simulink model "DCMachine"  (R2020a)
settings: Solver=VariableStepAuto  StartTime=0.0  StopTime=10.0  RelTol=1e-3
libraries: powerlib x4
settings Model: Creator=royde  LastModifiedBy=royde

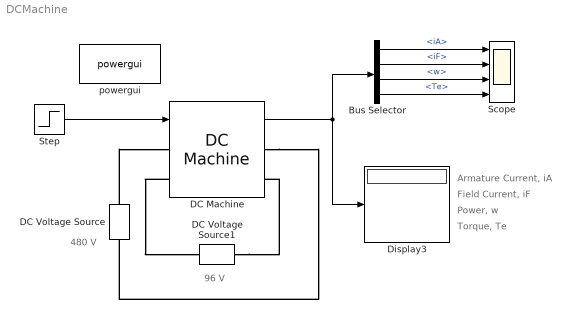
== system DCMachine ==
  note: Power, w
  note: Field Current, iF
  note: Armature Current, iA
  note: Torque, Te
  note: 96 V
  note: 480 V
  Bus Selector : BusSelector  OutputSignals=iA,iF,w,Te
  DC Machine : powerlib/Machines/DC Machine  PresetModel=03: 5HP 500V 1750RPM Field:300V  MechanicalLoad=Torque TL  FieldType=Wound  ShowDetailedParameters=on  MeasurementBus=on  RLa=[11.2 0.1215]  RLf=[281.3 156]  Laf=1.976  MachineConstant=Torque constant (N.m/A)  Ke=1.8  Kt=1.8  J=0.02215  Bm=0.002953  Tf=0.5161  w0=1  Ifinit=0.341272662637753  TsPowergui=0  TsBlock=-1
  DC Voltage Source : powerlib/Electrical Sources/DC Voltage Source  Amplitude=480  Measurements=None
  DC Voltage Source1 : powerlib/Electrical Sources/DC Voltage Source  Amplitude=96  Measurements=Voltage
  Display3 : Display
  Scope : Scope  NumInputPorts=4
  Step : Step  SampleTime=0
  powergui : powerlib/powergui  Priority=1  SimulationMode=Continuous  SampleTime=50e-6  frequency=60  Iterations=50  frequencyindice=0  Pbase=100e6  ErrMax=1e-4  UnitsV=kV  UnitsW=MW  buscounter=0  FunctionMessages=off  echomessages=off  EnableUseOfTLC=off  CurrentSourceSwitches=off  DisableSnubberDevices=off  DisableRonSwitches=off  DisableVfSwitches=off  DisplayEquations=off  AutomaticDiscreteSolvers=off  SolverType=Tustin/Backward Euler (TBE)  Interpol=off  ExternalGateDelay=off  methode=off  Ts=100  x0status=blocks  SPID=on  SwTol=0  HookPort=off  NonlinearTolerance=1e-4  nMaxIteration=100  ContinueOnMaxIteration=off  RestoreLinks=warning  ResistiveCurrentMeasurement=off  Frange=[0:2:500]  Ylog=off  Xlog=on  ShowGrid=off  save=off  variable=ZData  structure=0  ZoomFFT=off  StartTime=0.0  cycles=1  DisplayStyle=1  fundamental=60  FreqAxis=off  MaxFrequency=1000  frequencyindicesteady=1  RmsSteady=1  display=off
  wires:
  Step/1 -> DC Machine/1
  DC Machine/1 -> Display3/1, Bus Selector/1
  Bus Selector/1 -> Scope/1  "<iA>"
  Bus Selector/2 -> Scope/2  "<iF>"
  Bus Selector/3 -> Scope/3  "<w>"
  Bus Selector/4 -> Scope/4  "<Te>"
  connections:
  DC Machine/LConn2 -- DC Voltage Source1/RConn1
  DC Voltage Source1/LConn1 -- DC Machine/RConn2
  DC Voltage Source/RConn1 -- DC Machine/LConn1
  DC Machine/RConn1 -- DC Voltage Source/LConn1
